simulink model "lab3m1"  (R2018a)
settings: Solver=ode4  StartTime=0.0  StopTime=1  FixedStep=1e-2  RelTol=1e-3
values from neighbouring files (symbols this model uses):
  lambda = lambdas(i)    [MarcinGrzybSkrypt.m]
  stime = 0.1    [MarcinGrzybSkrypt.m]
  WPC = 0.5    [MarcinGrzybSkrypt.m]
settings Model: Creator=nicra  LastModifiedBy=nicra

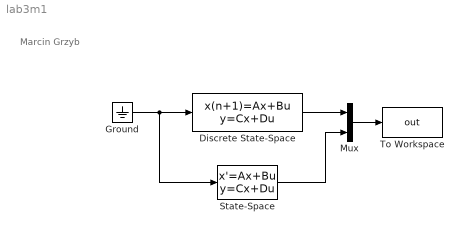
== system lab3m1 ==
  note: Marcin Grzyb
  Discrete State-Space : DiscreteStateSpace  A=lambda  B=0  D=0  InitialCondition=WPC  SampleTime=stime
  Ground : Ground
  Mux : Mux  Inputs=2
  State-Space : StateSpace  A=lambda  B=0  D=0  InitialCondition=WPC
  To Workspace : ToWorkspace  VariableName=out  SampleTime=-1
  wires:
  Ground/1 -> State-Space/1, Discrete State-Space/1
  Mux/1 -> To Workspace/1
  Discrete State-Space/1 -> Mux/1
  State-Space/1 -> Mux/2
